simulink library "PhD_Library"  (R2018a)
settings: Solver=VariableStepAuto  StartTime=0.0  StopTime=10.0  RelTol=1e-3
values from neighbouring files (symbols this model uses):
  Ts = Ts_c    (= 1e-07)    [PlantStateEquations_abc_Script.m]
undefined symbols (not defined in the file or in its folder): D1, Delta, DiscIntNeverNeededParam, ESS, f_LPF_noise, fcutouti, fcutoutv, fn, fsw, Iap, Kp, PCC, Sn, tctrl, Ti, Ts_control, Ts_PWM, Uabp, Uanp, WT, X, zeta
libraries: $bdroot x84, powerlib_meascontrol x59, powerlib x56, peTransforms x32, cstblocks x2, simulink x2
(part 2 of 5)

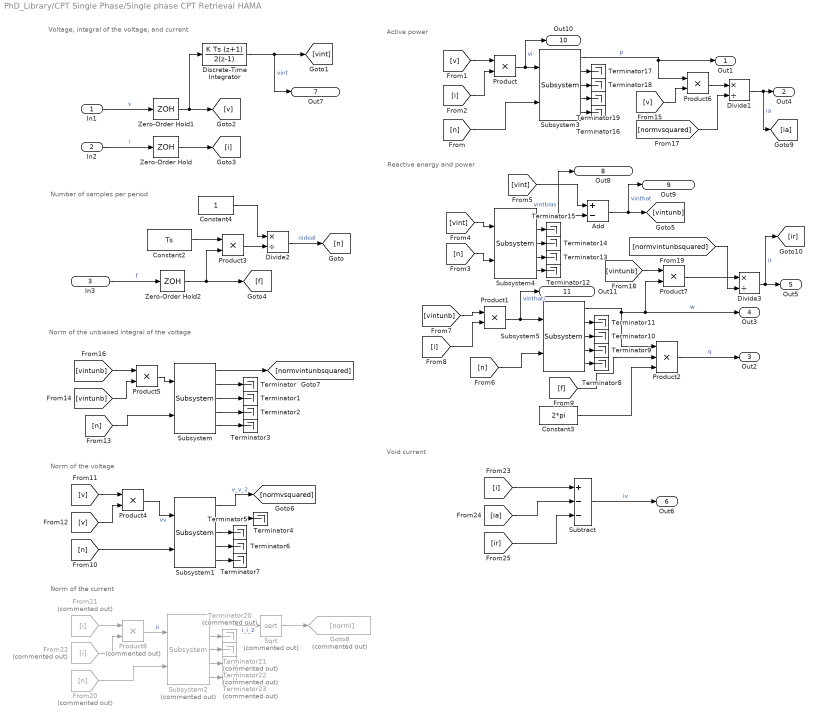
== system PhD_Library/CPT Single Phase/Single phase CPT Retrieval HAMA ==
  note: Void current
  note: Number of samples per period
  note: Norm of the voltage
  note: Voltage, integral of the voltage, and current
  note: Reactive energy and power
  note: Active power
  note: Norm of the current
  note: Norm of the unbiased integral of the voltage
  In1 : Inport
  In2 : Inport  Port=2
  In3 : Inport  Port=3
  Add : Sum  Inputs=+-
  Constant2 : Constant  Value=Ts
  Constant3 : Constant  Value=2*pi
  Constant4 : Constant
  Discrete-Time Integrator : DiscreteIntegrator  IntegratorMethod=Integration: Trapezoidal  SampleTime=Ts  ICPrevOutput=DiscIntNeverNeededParam  ICPrevScaledInput=DiscIntNeverNeededParam
  Divide1 : Product  Inputs=*/
  Divide2 : Product  Inputs=*/
  Divide3 : Product  Inputs=*/
  From20 : From  Commented=on  GotoTag=n
  From21 : From  Commented=on  GotoTag=i
  From22 : From  Commented=on  GotoTag=i
  Goto8 : Goto  Commented=on  GotoTag=normi
  Product{,1,3..7} (7 alike) : Product
  Product2 : Product  Inputs=3
  Product8 : Product  Commented=on
  Sqrt : Sqrt  Commented=on  SaturateOnIntegerOverflow=on
  Subsystem{,1,3..5} (5 alike) : $bdroot/Adaptive Moving Averages/Subsystem  NbSize=NbSize  Ts=Ts
  Subsystem2 : $bdroot/Adaptive Moving Averages/Subsystem  Commented=on  NbSize=NbSize  Ts=Ts
  Subtract : Sum  Inputs=+--
  Terminator{,1..19} (20 alike) : Terminator
  Terminator{20..23} (4 alike) : Terminator  Commented=on
  Zero-Order Hold : ZeroOrderHold  SampleTime=Ts
  Zero-Order Hold1 : ZeroOrderHold  SampleTime=Ts
  Zero-Order Hold2 : ZeroOrderHold  SampleTime=Ts
  Out1 : Outport
  Out4 : Outport  Port=2
  Out2 : Outport  Port=3
  Out3 : Outport  Port=4
  Out5 : Outport  Port=5
  Out6 : Outport  Port=6
  Out7 : Outport  Port=7
  Out8 : Outport  Port=8
  Out9 : Outport  Port=9
  Out10 : Outport  Port=10
  Out11 : Outport  Port=11
  wires:
  Product6/1 -> Divide1/1
  [i] -> Product/2
  Product3/1 -> Divide2/2
  Product7/1 -> Divide3/1
  [ia] -> Subtract/2
  [f] -> Product2/2
  Divide3/1 -> [ir], Out5/1  "ir"
  Subsystem2/1 -> Sqrt/1  "i_i_2"
  Product8/1 -> Subsystem2/1  "ii"
  [v] -> Product4/1
  Subtract/1 -> Out6/1  "iv"
  In2/1 -> Zero-Order Hold/1  "i"
  In1/1 -> Zero-Order Hold1/1  "v"
  [v] -> Product/1
  [v] -> Product4/2
  [n] -> Subsystem/2
  [vint] -> Add/1
  Add/1 -> Out9/1, [vintunb]  "vinthat"
  From21/1 -> Product8/1
  Subsystem4/1 -> Out8/1, Add/2  "vintbias"
  Zero-Order Hold2/1 -> Product3/2, [f]
  [ir] -> Subtract/3
  Divide2/1 -> [n]  "nideal"
  Product1/1 -> Subsystem5/1, Out11/1  "vinthati"
  Zero-Order Hold/1 -> [i]
  Divide1/1 -> [ia], Out4/1  "ia"
  [vintunb] -> Product7/1
  Product2/1 -> Out2/1  "q"
  Constant3/1 -> Product2/3
  From22/1 -> Product8/2
  [vintunb] -> Product5/1
  [normvintunbsquared] -> Divide3/2
  Discrete-Time Integrator/1 -> Out7/1, [vint]  "vint"
  [vintunb] -> Product5/2
  [i] -> Subtract/1
  Product5/1 -> Subsystem/1
  [vintunb] -> Product1/1
  Subsystem1/1 -> [normvsquared]  "v_v_2"
  Product/1 -> Subsystem3/1, Out10/1  "vi"
  [v] -> Product6/2
  Constant2/1 -> Product3/1
  [i] -> Product1/2
  Product4/1 -> Subsystem1/1  "vv"
  [n] -> Subsystem1/2
  Subsystem5/1 -> Product2/1, Product7/2, Out3/1  "w"
  [normvsquared] -> Divide1/2
  Zero-Order Hold1/1 -> [v], Discrete-Time Integrator/1
  In3/1 -> Zero-Order Hold2/1  "f"
  Constant4/1 -> Divide2/1
  Subsystem/1 -> [normvintunbsquared]
  Sqrt/1 -> Goto8/1
  Subsystem3/1 -> Product6/1, Out1/1  "p"
  From20/1 -> Subsystem2/2
  [n] -> Subsystem3/2
  [vint] -> Subsystem4/1
  [n] -> Subsystem4/2
  [n] -> Subsystem5/2
  Subsystem/2 -> Terminator/1
  Subsystem/3 -> Terminator1/1
  Subsystem/4 -> Terminator2/1
  Subsystem/5 -> Terminator3/1
  Subsystem1/2 -> Terminator4/1
  Subsystem1/3 -> Terminator5/1
  Subsystem1/4 -> Terminator6/1
  Subsystem1/5 -> Terminator7/1
  Subsystem5/5 -> Terminator8/1
  Subsystem5/4 -> Terminator9/1
  Subsystem5/3 -> Terminator10/1
  Subsystem5/2 -> Terminator11/1
  Subsystem4/5 -> Terminator12/1
  Subsystem4/4 -> Terminator13/1
  Subsystem4/3 -> Terminator14/1
  Subsystem4/2 -> Terminator15/1
  Subsystem3/5 -> Terminator16/1
  Subsystem3/2 -> Terminator17/1
  Subsystem3/3 -> Terminator18/1
  Subsystem3/4 -> Terminator19/1
  Subsystem2/2 -> Terminator20/1
  Subsystem2/3 -> Terminator21/1
  Subsystem2/4 -> Terminator22/1
  Subsystem2/5 -> Terminator23/1

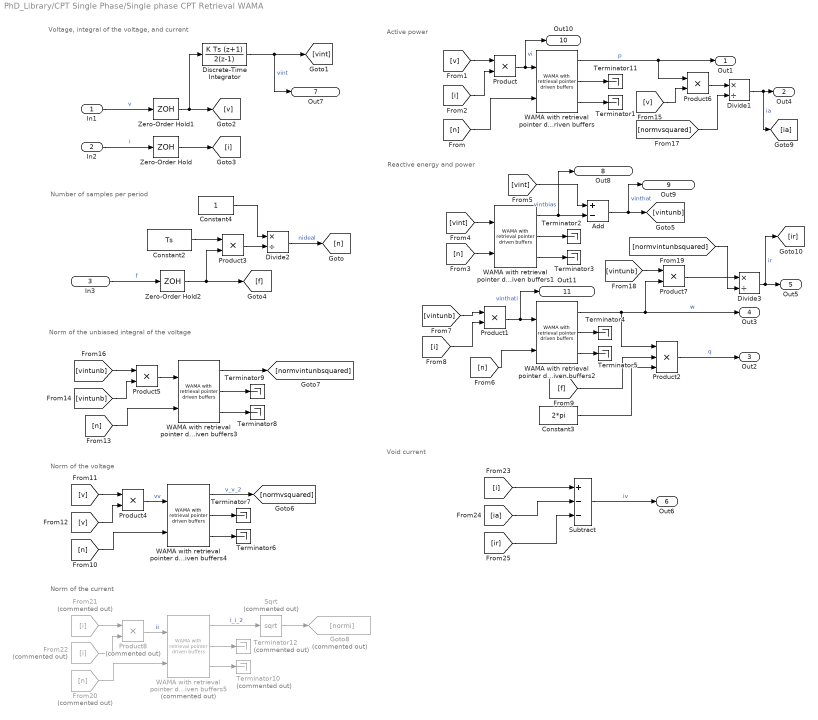
== system PhD_Library/CPT Single Phase/Single phase CPT Retrieval WAMA ==
  note: Voltage, integral of the voltage, and current
  note: Number of samples per period
  note: Reactive energy and power
  note: Active power
  note: Norm of the voltage
  note: Norm of the unbiased integral of the voltage
  note: Norm of the current
  note: Void current
  In1 : Inport
  In2 : Inport  Port=2
  In3 : Inport  Port=3
  Add : Sum  Inputs=+-
  Constant2 : Constant  Value=Ts
  Constant3 : Constant  Value=2*pi
  Constant4 : Constant
  Discrete-Time Integrator : DiscreteIntegrator  IntegratorMethod=Integration: Trapezoidal  SampleTime=Ts  ICPrevOutput=DiscIntNeverNeededParam  ICPrevScaledInput=DiscIntNeverNeededParam
  Divide1 : Product  Inputs=*/
  Divide2 : Product  Inputs=*/
  Divide3 : Product  Inputs=*/
  From20 : From  Commented=on  GotoTag=n
  From21 : From  Commented=on  GotoTag=i
  From22 : From  Commented=on  GotoTag=i
  Goto8 : Goto  Commented=on  GotoTag=normi
  Product{,1,3..7} (7 alike) : Product
  Product2 : Product  Inputs=3
  Product8 : Product  Commented=on
  Sqrt : Sqrt  Commented=on  SaturateOnIntegerOverflow=on
  Subtract : Sum  Inputs=+--
  Terminator{1..9,11} (10 alike) : Terminator
  Terminator10 : Terminator  Commented=on
  Terminator12 : Terminator  Commented=on
  WAMA with retrieval pointer driven buffers{,1..4} (5 alike) : $bdroot/Adaptive Moving Averages/WAMA with retrieval pointer driven buffers  NbSize=NbSize  Ts=Ts
  WAMA with retrieval pointer driven buffers5 : $bdroot/Adaptive Moving Averages/WAMA with retrieval pointer driven buffers  Commented=on  NbSize=NbSize  Ts=Ts
  Zero-Order Hold : ZeroOrderHold  SampleTime=Ts
  Zero-Order Hold1 : ZeroOrderHold  SampleTime=Ts
  Zero-Order Hold2 : ZeroOrderHold  SampleTime=Ts
  Out1 : Outport
  Out4 : Outport  Port=2
  Out2 : Outport  Port=3
  Out3 : Outport  Port=4
  Out5 : Outport  Port=5
  Out6 : Outport  Port=6
  Out7 : Outport  Port=7
  Out8 : Outport  Port=8
  Out9 : Outport  Port=9
  Out10 : Outport  Port=10
  Out11 : Outport  Port=11
  wires:
  Discrete-Time Integrator/1 -> Out7/1, [vint]  "vint"
  In3/1 -> Zero-Order Hold2/1  "f"
  Zero-Order Hold1/1 -> [v], Discrete-Time Integrator/1
  [i] -> Subtract/1
  WAMA with retrieval pointer driven buffers3/1 -> [normvintunbsquared]
  Product5/1 -> WAMA with retrieval pointer driven buffers3/1
  WAMA with retrieval pointer driven buffers3/2 -> Terminator9/1
  WAMA with retrieval pointer driven buffers3/3 -> Terminator8/1
  Product4/1 -> WAMA with retrieval pointer driven buffers4/1  "vv"
  WAMA with retrieval pointer driven buffers4/3 -> Terminator6/1
  WAMA with retrieval pointer driven buffers4/2 -> Terminator7/1
  WAMA with retrieval pointer driven buffers4/1 -> [normvsquared]  "v_v_2"
  [n] -> WAMA with retrieval pointer driven buffers4/2
  [vint] -> WAMA with retrieval pointer driven buffers1/1
  WAMA with retrieval pointer driven buffers5/3 -> Terminator10/1
  WAMA with retrieval pointer driven buffers1/2 -> Terminator2/1
  WAMA with retrieval pointer driven buffers/2 -> Terminator11/1
  WAMA with retrieval pointer driven buffers/3 -> Terminator1/1
  WAMA with retrieval pointer driven buffers2/2 -> Terminator4/1
  Product1/1 -> Out11/1, WAMA with retrieval pointer driven buffers2/1  "vinthati"
  [v] -> Product6/2
  WAMA with retrieval pointer driven buffers2/1 -> Product7/2, Out3/1, Product2/1  "w"
  Product/1 -> Out10/1, WAMA with retrieval pointer driven buffers/1  "vi"
  [vintunb] -> Product7/1
  [normvsquared] -> Divide1/2
  [normvintunbsquared] -> Divide3/2
  Divide1/1 -> [ia], Out4/1  "ia"
  Zero-Order Hold/1 -> [i]
  [vint] -> Add/1
  Constant3/1 -> Product2/3
  [i] -> Product1/2
  [vintunb] -> Product1/1
  Constant2/1 -> Product3/1
  [vintunb] -> Product5/1
  [ir] -> Subtract/3
  From22/1 -> Product8/2
  [n] -> WAMA with retrieval pointer driven buffers2/2
  WAMA with retrieval pointer driven buffers5/2 -> Terminator12/1
  Zero-Order Hold2/1 -> Product3/2, [f]
  Product7/1 -> Divide3/1
  WAMA with retrieval pointer driven buffers1/3 -> Terminator3/1
  Sqrt/1 -> Goto8/1
  Divide2/1 -> [n]  "nideal"
  WAMA with retrieval pointer driven buffers5/1 -> Sqrt/1  "i_i_2"
  Constant4/1 -> Divide2/1
  Product2/1 -> Out2/1  "q"
  [n] -> WAMA with retrieval pointer driven buffers3/2
  Product3/1 -> Divide2/2
  [n] -> WAMA with retrieval pointer driven buffers/2
  From20/1 -> WAMA with retrieval pointer driven buffers5/2
  [vintunb] -> Product5/2
  [v] -> Product4/2
  Product8/1 -> WAMA with retrieval pointer driven buffers5/1  "ii"
  Product6/1 -> Divide1/1
  WAMA with retrieval pointer driven buffers1/1 -> Out8/1, Add/2  "vintbias"
  Add/1 -> Out9/1, [vintunb]  "vinthat"
  [f] -> Product2/2
  In1/1 -> Zero-Order Hold1/1  "v"
  From21/1 -> Product8/1
  WAMA with retrieval pointer driven buffers/1 -> Product6/1, Out1/1  "p"
  Subtract/1 -> Out6/1  "iv"
  [i] -> Product/2
  In2/1 -> Zero-Order Hold/1  "i"
  [n] -> WAMA with retrieval pointer driven buffers1/2
  Divide3/1 -> [ir], Out5/1  "ir"
  [v] -> Product4/1
  WAMA with retrieval pointer driven buffers2/3 -> Terminator5/1
  [v] -> Product/1
  [ia] -> Subtract/2

== system PhD_Library/Offshore_Oil_and_Wind/Balanced_3_phase_Vsource ==
  amp_pu : Inport
  time_s : Inport  Port=2
  phase_deg : Inport  Port=3
  pos1_neg-1 : Inport  Port=4
  f_pu : Inport  Port=5
  Add3 : Sum  Inputs=+-+
  Add4 : Sum  Inputs=+++
  Add5 : Sum
  Amplitude_Base : Constant  Value=BaseAmp
  Bus Creator : BusCreator  Inputs=3
  Constant : Constant  Value=2*pi
  Constant4 : Constant  Value=2*pi/3
  Constant6 : Constant  Value=2*pi
  Controlled Voltage Source : powerlib/Electrical Sources/Controlled Voltage Source  Initialize=off  Source_Type=AC  Amplitude=ESS.LSC.Ub*(2/3)^0.5  Phase=0  Frequency=PCC.fn  Measurements=None
  Controlled Voltage Source1 : powerlib/Electrical Sources/Controlled Voltage Source  Initialize=off  Source_Type=AC  Amplitude=ESS.LSC.Ub*(2/3)^0.5  Phase=-120  Frequency=PCC.fn  Measurements=None
  Controlled Voltage Source2 : powerlib/Electrical Sources/Controlled Voltage Source  Initialize=off  Source_Type=AC  Amplitude=ESS.LSC.Ub*(2/3)^0.5  Phase=120  Frequency=PCC.fn  Measurements=None
  Gain : Gain  Gain=pi/180
  Gain1 : Gain  Gain=fn
  Mux : Mux  Inputs=3
  Product{1,3..8} (7 alike) : Product
  Product2 : Product  Inputs=3
  Relay : Relay  OnSwitchValue=0  OffSwitchValue=-0.1  OffOutputValue=-1
  Trigonometric Function3 : Trigonometry
  Trigonometric Function4 : Trigonometry
  Trigonometric Function5 : Trigonometry
  mod : Math  Operator=mod  SaturateOnIntegerOverflow=on
  Va+ : PMIOPort  Side=Right
  Vb+ : PMIOPort  Port=2  Side=Right
  Vc+ : PMIOPort  Port=3  Side=Right
  Va- : PMIOPort  Port=4  Side=Right
  Vb- : PMIOPort  Port=5  Side=Right
  Vc- : PMIOPort  Port=6  Side=Right
  Amp_V : Outport
  phase_rad : Outport  Port=2
  wt_phase_abc : Outport  Port=3
  Vabc : Outport  Port=4
  wires:
  Add4/1 -> Mux/3, Trigonometric Function5/1
  Product6/1 -> phase_rad/1, Add4/3, Add3/3, Add5/2  "phase"
  Add3/1 -> Mux/2, Trigonometric Function4/1
  pos1_neg-1/1 -> Relay/1
  Product3/1 -> Bus Creator/1, Controlled Voltage Source/1  "Va"
  amp_pu/1 -> Product1/1
  Product8/1 -> Add3/2, Add4/2
  Product5/1 -> Bus Creator/3, Controlled Voltage Source2/1  "Vc"
  Product4/1 -> Bus Creator/2, Controlled Voltage Source1/1  "Vb"
  Amplitude_Base/1 -> Product1/2
  Product7/1 -> Product8/1
  Product1/1 -> Product5/1, Product4/1, Product3/1, Amp_V/1  "amp"
  Relay/1 -> Product8/2
  Trigonometric Function3/1 -> Product3/2
  Product2/1 -> Add5/1, Add4/1, Add3/1  "wt"
  Trigonometric Function5/1 -> Product5/2
  Add5/1 -> Mux/1, Trigonometric Function3/1
  Trigonometric Function4/1 -> Product4/2
  phase_deg/1 -> Gain/1
  time_s/1 -> Product2/2
  Constant/1 -> Product2/1
  Gain1/1 -> Product2/3
  Bus Creator/1 -> Vabc/1
  Constant6/1 -> mod/2
  mod/1 -> wt_phase_abc/1
  Gain/1 -> Product6/1  "phase"
  Constant4/1 -> Product7/2
  Mux/1 -> mod/1
  f_pu/1 -> Product7/1, Product6/2, Gain1/1
  connections:
  Vb+/RConn1 -- Controlled Voltage Source1/RConn1
  Vc+/RConn1 -- Controlled Voltage Source2/RConn1
  Va+/RConn1 -- Controlled Voltage Source/RConn1
  Va-/RConn1 -- Controlled Voltage Source/LConn1
  Vb-/RConn1 -- Controlled Voltage Source1/LConn1
  Vc-/RConn1 -- Controlled Voltage Source2/LConn1

== system PhD_Library/Offshore_Oil_and_Wind/Digital first order LPF ==
  note: Transfer function: alpha / ( 1 + ( alpha -1 ) z^{-1} )
  note: alpha = Ts / ( 1/(2 pi fcutout) + Ts )
  note: y = alpha x + ( 1 - alpha) y z^{-1}
  in : Inport
  Add7 : Sum  Commented=on  Inputs=+-
  Discrete Filter : DiscreteFilter  Numerator=[Ts/(1/(2*pi*fcutout)+Ts)]  Denominator=[1 Ts/(1/(2*pi*fcutout)+Ts)-1]  SampleTime=Ts
  Discrete-Time Integrator : DiscreteIntegrator  Commented=on  IntegratorMethod=Integration: Trapezoidal  SampleTime=Ts  ICPrevOutput=DiscIntNeverNeededParam  ICPrevScaledInput=DiscIntNeverNeededParam
  Gain6 : Gain  Commented=on  Gain=2*pi*fcutout
  Rate Transition3 : RateTransition  OutPortSampleTime=Ts
  out : Outport
  wires:
  Add7/1 -> Gain6/1
  Discrete-Time Integrator/1 -> Add7/2
  in/1 -> Rate Transition3/1
  Gain6/1 -> Discrete-Time Integrator/1
  Rate Transition3/1 -> Add7/1, Discrete Filter/1
  Discrete Filter/1 -> out/1

== system PhD_Library/Offshore_Oil_and_Wind/DualRegulator ==
  idqref : Inport
  vabc : Inport  Port=2
  iabc : Inport  Port=3
  wt : Inport  Port=4
  w_pu : Inport  Port=5
  Udc : Inport  Port=6
  1=enable_acb : Inport  Port=7
  1=no,2=Notch,3=DSC : Inport  Port=8
  pre_mult_PI_errors : Inport  Port=9
  force_int : Inport  Port=10
  force_val : Inport  Port=11
  Bus Creator : BusCreator  Inputs=4
  Constant1 : Constant  Value=0
  Constant10 : Constant
  Constant14 : Constant
  Constant18 : Constant  Value=[0 0]
  Constant6 : Constant
  Constant8 : Constant  Value=0
  Idq_Dec_Signs_Fdbk_Ref : $bdroot/Offshore_Oil_and_Wind/Idq_Dec_Signs_Fdbk_Ref  Ts=Ts  fn=fgrid  Kp=PI_Kp  Ti=PI_Ti  L=PI_X  PI_max=PI_max  PI_min=PI_min  TrafoPhaseComp=0
  Idq_Dec_Signs_Fdbk_Ref_acb : $bdroot/Offshore_Oil_and_Wind/Idq_Dec_Signs_Fdbk_Ref  Ts=Ts  fn=fgrid  Kp=PI_Kp  Ti=PI_Ti  L=PI_X  PI_max=PI_max  PI_min=PI_min  TrafoPhaseComp=0
  PWM_abc_negwt_acb : $bdroot/Offshore_Oil_and_Wind/PWM_abc_negwt_acb  fsw=PWM_fsw  Ts=PWM_Ts  Uabp=PWM_Uabp  PWM_Ini_Phase=PWM_Ini
  Selector1 : Selector  InputPortWidth=3  IndexOptions=Index vector (dialog)  Indices=[1 3 2]  OutputSizes=1
  Selector7 : Selector  InputPortWidth=3  IndexOptions=Index vector (dialog)  Indices=[1 3 2]  OutputSizes=1
  Terminator{1..4,24} (5 alike) : Terminator
  abc_dq_bypassnotch : $bdroot/Offshore_Oil_and_Wind/abc_dq_bypassnotch  Ts=Ts  fn=2*fgrid  fcutoutv=fcutoutLPF  fcutouti=fcutoutLPF  zeta=zetanotch
  abc_dq_bypassnotch1 : $bdroot/Offshore_Oil_and_Wind/abc_dq_bypassnotch  Ts=Ts  fn=2*fgrid  fcutoutv=fcutoutLPF  fcutouti=fcutoutLPF  zeta=zetanotch
  idqref_gen_for_cnst_p : $bdroot/Offshore_Oil_and_Wind/idqref_gen_for_cnst_p  Ts_control=Ts
  PWMpulses : Outport
  Uabcref : Outport  Port=2
  mvidq : Outport  Port=3
  mpi+ : Outport  Port=4
  mpi- : Outport  Port=5
  wires:
  Udc/1 -> PWM_abc_negwt_acb/7
  abc_dq_bypassnotch1/1 -> idqref_gen_for_cnst_p/2, Bus Creator/3, Idq_Dec_Signs_Fdbk_Ref_acb/2  "vdq-"
  [w_pu] -> Idq_Dec_Signs_Fdbk_Ref/4
  PWM_abc_negwt_acb/3 -> Terminator24/1
  Constant14/1 -> Idq_Dec_Signs_Fdbk_Ref_acb/5
  abc_dq_bypassnotch/1 -> idqref_gen_for_cnst_p/1, Bus Creator/1, Idq_Dec_Signs_Fdbk_Ref/2  "vdq+"
  abc_dq_bypassnotch1/2 -> Bus Creator/4, Idq_Dec_Signs_Fdbk_Ref_acb/3  "idq-"
  Constant10/1 -> PWM_abc_negwt_acb/2
  Constant8/1 -> PWM_abc_negwt_acb/4
  abc_dq_bypassnotch/2 -> Bus Creator/2, Idq_Dec_Signs_Fdbk_Ref/3  "idq+"
  1=enable_acb/1 -> PWM_abc_negwt_acb/6
  Idq_Dec_Signs_Fdbk_Ref/1 -> PWM_abc_negwt_acb/1
  PWM_abc_negwt_acb/1 -> PWMpulses/1
  PWM_abc_negwt_acb/2 -> Uabcref/1  "Uabcref"
  Constant6/1 -> Idq_Dec_Signs_Fdbk_Ref/5
  Constant1/1 -> Idq_Dec_Signs_Fdbk_Ref_acb/6, Idq_Dec_Signs_Fdbk_Ref/6
  vabc/1 -> abc_dq_bypassnotch/1, Selector7/1
  iabc/1 -> abc_dq_bypassnotch/2, Selector1/1
  Idq_Dec_Signs_Fdbk_Ref_acb/1 -> PWM_abc_negwt_acb/5
  wt/1 -> abc_dq_bypassnotch/3, abc_dq_bypassnotch1/3, [theta]
  Selector7/1 -> abc_dq_bypassnotch1/1
  Selector1/1 -> abc_dq_bypassnotch1/2
  Constant18/1 -> PWM_abc_negwt_acb/3
  idqref/1 -> idqref_gen_for_cnst_p/3, Idq_Dec_Signs_Fdbk_Ref/1
  idqref_gen_for_cnst_p/1 -> Idq_Dec_Signs_Fdbk_Ref_acb/1
  [theta] -> PWM_abc_negwt_acb/8
  1=no,2=Notch,3=DSC/1 -> abc_dq_bypassnotch/5, abc_dq_bypassnotch1/5
  Bus Creator/1 -> mvidq/1
  w_pu/1 -> abc_dq_bypassnotch/4, abc_dq_bypassnotch1/4, [w_pu]
  [w_pu] -> Idq_Dec_Signs_Fdbk_Ref_acb/4
  pre_mult_PI_errors/1 -> Idq_Dec_Signs_Fdbk_Ref_acb/7, Idq_Dec_Signs_Fdbk_Ref/7
  force_int/1 -> Idq_Dec_Signs_Fdbk_Ref_acb/8, Idq_Dec_Signs_Fdbk_Ref/8
  force_val/1 -> Idq_Dec_Signs_Fdbk_Ref_acb/10, Idq_Dec_Signs_Fdbk_Ref_acb/9, Idq_Dec_Signs_Fdbk_Ref/10, Idq_Dec_Signs_Fdbk_Ref/9
  Idq_Dec_Signs_Fdbk_Ref/4 -> mpi+/1
  Idq_Dec_Signs_Fdbk_Ref_acb/4 -> mpi-/1
  Idq_Dec_Signs_Fdbk_Ref/2 -> Terminator1/1
  Idq_Dec_Signs_Fdbk_Ref/3 -> Terminator2/1
  Idq_Dec_Signs_Fdbk_Ref_acb/2 -> Terminator3/1
  Idq_Dec_Signs_Fdbk_Ref_acb/3 -> Terminator4/1

== system PhD_Library/Offshore_Oil_and_Wind/Enabled ==
  En : Inport
  MATLAB Function : MATLAB Function  SystemSampleTime=Ts
      settings: RTWSystemCode=Inline
  Enabled : Outport
  Disabled : Outport  Port=2
  wires:
  En/1 -> MATLAB Function/1(En)
  MATLAB Function/1(Enabled) -> Enabled/1
  MATLAB Function/2(Disabled) -> Disabled/1

== system PhD_Library/Offshore_Oil_and_Wind/Garbage ==
  In1 : Inport
  In2 : Inport  Port=2
  Demux4 : Demux  Outputs=3
  Demux5 : Demux  Outputs=3
  Mux3 : Mux  Inputs=[1 1 1]
  Mux4 : Mux  Inputs=[1 1 1]
  Transfer Fcn : TransferFcn  Denominator=[1/(2*pi*fcutoutv) 1]
  Transfer Fcn1 : TransferFcn  Denominator=[1/(2*pi*fcutoutv) 1]
  Transfer Fcn2 : TransferFcn  Denominator=[1/(2*pi*fcutoutv) 1]
  Transfer Fcn3 : TransferFcn  Denominator=[1/(2*pi*fcutouti) 1]
  Transfer Fcn4 : TransferFcn  Denominator=[1/(2*pi*fcutouti) 1]
  Transfer Fcn5 : TransferFcn  Denominator=[1/(2*pi*fcutouti) 1]
  Out1 : Outport
  Out2 : Outport  Port=2
  wires:
  Demux5/1 -> Transfer Fcn3/1
  Transfer Fcn2/1 -> Mux3/3
  Demux4/1 -> Transfer Fcn/1
  Demux5/3 -> Transfer Fcn5/1
  Transfer Fcn3/1 -> Mux4/1
  Transfer Fcn4/1 -> Mux4/2
  Demux4/3 -> Transfer Fcn2/1
  Transfer Fcn5/1 -> Mux4/3
  Demux4/2 -> Transfer Fcn1/1
  Transfer Fcn/1 -> Mux3/1
  Mux3/1 -> Out2/1
  Transfer Fcn1/1 -> Mux3/2
  Demux5/2 -> Transfer Fcn4/1
  In1/1 -> Demux5/1
  Mux4/1 -> Out1/1
  In2/1 -> Demux4/1

== system PhD_Library/Offshore_Oil_and_Wind/Ideal3PhaseVoltSource ==
  amp_pu : Inport
  f_pu : Inport  Port=2
  phase_deg : Inport  Port=3
  pos1_neg-1 : Inport  Port=4
  Harm_nr : Inport  Port=5
  Add3 : Sum  Inputs=+-+
  Add4 : Sum  Inputs=+++
  Add5 : Sum
  Amplitude_Base : Constant  Value=BaseAmp
  Bus Creator : BusCreator  Inputs=3
  Constant : Constant  Value=2*pi
  Constant4 : Constant  Value=2*pi/3
  Constant6 : Constant  Value=2*pi
  Controlled Voltage Source : powerlib/Electrical Sources/Controlled Voltage Source  Initialize=off  Source_Type=AC  Amplitude=ESS.LSC.Ub*(2/3)^0.5  Phase=0  Frequency=PCC.fn  Measurements=None
  Controlled Voltage Source1 : powerlib/Electrical Sources/Controlled Voltage Source  Initialize=off  Source_Type=AC  Amplitude=ESS.LSC.Ub*(2/3)^0.5  Phase=-120  Frequency=PCC.fn  Measurements=None
  Controlled Voltage Source2 : powerlib/Electrical Sources/Controlled Voltage Source  Initialize=off  Source_Type=AC  Amplitude=ESS.LSC.Ub*(2/3)^0.5  Phase=120  Frequency=PCC.fn  Measurements=None
  Gain : Gain  Gain=pi/180
  Gain1 : Gain  Gain=fn
  Integrator : Integrator
  Mux : Mux  Inputs=3
  Product{1,3..8} (7 alike) : Product
  Product2 : Product  Inputs=3
  Relay : Relay  OnSwitchValue=0  OffSwitchValue=-0.1  OffOutputValue=-1
  Trigonometric Function3 : Trigonometry
  Trigonometric Function4 : Trigonometry
  Trigonometric Function5 : Trigonometry
  mod : Math  Operator=mod  SaturateOnIntegerOverflow=on
  Va+ : PMIOPort  Side=Right
  Vb+ : PMIOPort  Port=2  Side=Right
  Vc+ : PMIOPort  Port=3  Side=Right
  Va- : PMIOPort  Port=4  Side=Right
  Vb- : PMIOPort  Port=5  Side=Right
  Vc- : PMIOPort  Port=6  Side=Right
  Amp_V : Outport
  phase_rad : Outport  Port=2
  wt_phase_abc : Outport  Port=3
  Vabc : Outport  Port=4
  wires:
  Add4/1 -> Mux/3, Trigonometric Function5/1
  Product6/1 -> phase_rad/1, Add4/3, Add3/3, Add5/2  "phase"
  Add3/1 -> Mux/2, Trigonometric Function4/1
  pos1_neg-1/1 -> Relay/1
  Product3/1 -> Bus Creator/1, Controlled Voltage Source/1  "Va"
  amp_pu/1 -> Product1/1
  Product8/1 -> Add3/2, Add4/2
  Product5/1 -> Bus Creator/3, Controlled Voltage Source2/1  "Vc"
  Product4/1 -> Bus Creator/2, Controlled Voltage Source1/1  "Vb"
  Amplitude_Base/1 -> Product1/2
  Product7/1 -> Product8/1
  Product1/1 -> Product5/1, Product4/1, Product3/1, Amp_V/1  "amp"
  Relay/1 -> Product8/2
  Trigonometric Function3/1 -> Product3/2
  Product2/1 -> Add5/1, Add4/1, Add3/1  "wt"
  Trigonometric Function5/1 -> Product5/2
  Add5/1 -> Mux/1, Trigonometric Function3/1
  Trigonometric Function4/1 -> Product4/2
  phase_deg/1 -> Gain/1
  f_pu/1 -> Integrator/1
  Constant/1 -> Product2/1
  Gain1/1 -> Product2/3
  Bus Creator/1 -> Vabc/1
  Constant6/1 -> mod/2
  mod/1 -> wt_phase_abc/1
  Gain/1 -> Product6/1  "phase"
  Constant4/1 -> Product7/2
  Mux/1 -> mod/1
  Harm_nr/1 -> Product7/1, Product6/2, Gain1/1
  Integrator/1 -> Product2/2  "time"
  connections:
  Vb+/RConn1 -- Controlled Voltage Source1/RConn1
  Vc+/RConn1 -- Controlled Voltage Source2/RConn1
  Va+/RConn1 -- Controlled Voltage Source/RConn1
  Va-/RConn1 -- Controlled Voltage Source/LConn1
  Vb-/RConn1 -- Controlled Voltage Source1/LConn1
  Vc-/RConn1 -- Controlled Voltage Source2/LConn1

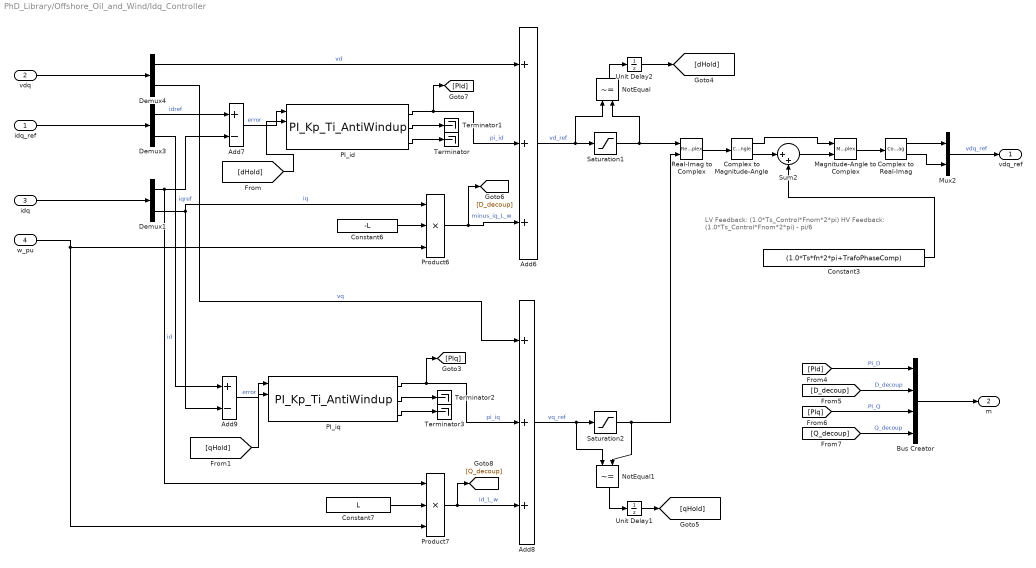
== system PhD_Library/Offshore_Oil_and_Wind/Idq_Controller ==
  note: LV Feedback: (1.0*Ts_Control*Fnom*2*pi)
      | HV Feedback: (1.0*Ts_Control*Fnom*2*pi) - pi/6
  idq_ref : Inport
  vdq : Inport  Port=2
  idq : Inport  Port=3
  w_pu : Inport  Port=4
  Add6 : Sum  Inputs=+++
  Add7 : Sum  Inputs=+-
  Add8 : Sum  Inputs=+++
  Add9 : Sum  Inputs=+-
  Bus Creator : BusCreator  Inputs=4
  Complex to Magnitude-Angle : ComplexToMagnitudeAngle
  Complex to Real-Imag : ComplexToRealImag
  Constant3 : Constant  Value=(1.0*Ts*fn*2*pi+TrafoPhaseComp)  SampleTime=Ts
  Constant6 : Constant  Value=-L  SampleTime=Ts
  Constant7 : Constant  Value=L  SampleTime=Ts
  Demux1 : Demux  Outputs=2
  Demux3 : Demux  Outputs=2
  Demux4 : Demux  Outputs=2
  Magnitude-Angle to Complex : MagnitudeAngleToComplex
  Mux2 : Mux  Inputs=2
  NotEqual : RelationalOperator  Operator=~=  OutDataTypeStr=boolean  RndMeth=Simplest
  NotEqual1 : RelationalOperator  Operator=~=  OutDataTypeStr=boolean  RndMeth=Simplest
  PI_id : $bdroot/Offshore_Oil_and_Wind/PI_Kp_Ti_AntiWindup  Ts=Ts  Kp=Kp  Ti=Ti  PI_max=PI_max  PI_min=PI_min
  PI_iq : $bdroot/Offshore_Oil_and_Wind/PI_Kp_Ti_AntiWindup  Ts=Ts  Kp=Kp  Ti=Ti  PI_max=PI_max  PI_min=PI_min
  Product6 : Product  Inputs=3  RndMeth=Zero
  Product7 : Product  Inputs=3  RndMeth=Zero
  Real-Imag to Complex : RealImagToComplex
  Saturation1 : Saturate  UpperLimit=PI_max  LowerLimit=PI_min
  Saturation2 : Saturate  UpperLimit=PI_max  LowerLimit=PI_min
  Sum2 : Sum  Inputs=|++
  Terminator{,1..3} (4 alike) : Terminator
  Unit Delay1 : UnitDelay  SampleTime=Ts
  Unit Delay2 : UnitDelay  SampleTime=Ts
  vdq_ref : Outport
  m : Outport  Port=2
  wires:
  PI_iq/1 -> [PIq], Add8/2  "pi_iq"
  PI_iq/2 -> Terminator2/1
  PI_id/2 -> Terminator1/1
  w_pu/1 -> Product7/3, Product6/3
  Add9/1 -> PI_iq/1  "error"
  PI_id/1 -> [PId], Add6/2  "pi_id"
  Constant6/1 -> Product6/2
  Constant7/1 -> Product7/2
  Demux1/1 -> Add7/2, Product7/1  "id"
  Product7/1 -> [Q_decoup], Add8/3  "id_L_w"
  Demux4/1 -> Add6/1  "vd"
  Add7/1 -> PI_id/1  "error"
  Demux1/2 -> Product6/1, Add9/2  "iq"
  Product6/1 -> [D_decoup], Add6/3  "minus_iq_L_w"
  PI_iq/3 -> Terminator3/1
  PI_id/3 -> Terminator/1
  Demux4/2 -> Add8/1  "vq"
  Mux2/1 -> vdq_ref/1  "vdq_ref"
  idq/1 -> Demux1/1
  vdq/1 -> Demux4/1
  Add8/1 -> NotEqual1/1, Saturation2/1  "vq_ref"
  Add6/1 -> NotEqual/1, Saturation1/1  "vd_ref"
  idq_ref/1 -> Demux3/1
  Demux3/1 -> Add7/1  "idref"
  Demux3/2 -> Add9/1  "iqref"
  Magnitude-Angle to Complex/1 -> Complex to Real-Imag/1
  Real-Imag to Complex/1 -> Complex to Magnitude-Angle/1
  Complex to Magnitude-Angle/1 -> Magnitude-Angle to Complex/1
  Complex to Magnitude-Angle/2 -> Sum2/1
  Sum2/1 -> Magnitude-Angle to Complex/2
  Constant3/1 -> Sum2/2
  Complex to Real-Imag/1 -> Mux2/1
  Complex to Real-Imag/2 -> Mux2/2
  [PId] -> Bus Creator/1  "PI_D"
  [D_decoup] -> Bus Creator/2  "D_decoup"
  [PIq] -> Bus Creator/3  "PI_Q"
  Bus Creator/1 -> m/1
  [Q_decoup] -> Bus Creator/4  "Q_decoup"
  Saturation1/1 -> NotEqual/2, Real-Imag to Complex/1
  NotEqual/1 -> Unit Delay2/1
  Saturation2/1 -> NotEqual1/2, Real-Imag to Complex/2
  NotEqual1/1 -> Unit Delay1/1
  Unit Delay2/1 -> [dHold]
  Unit Delay1/1 -> [qHold]
  [dHold] -> PI_id/2
  [qHold] -> PI_iq/2

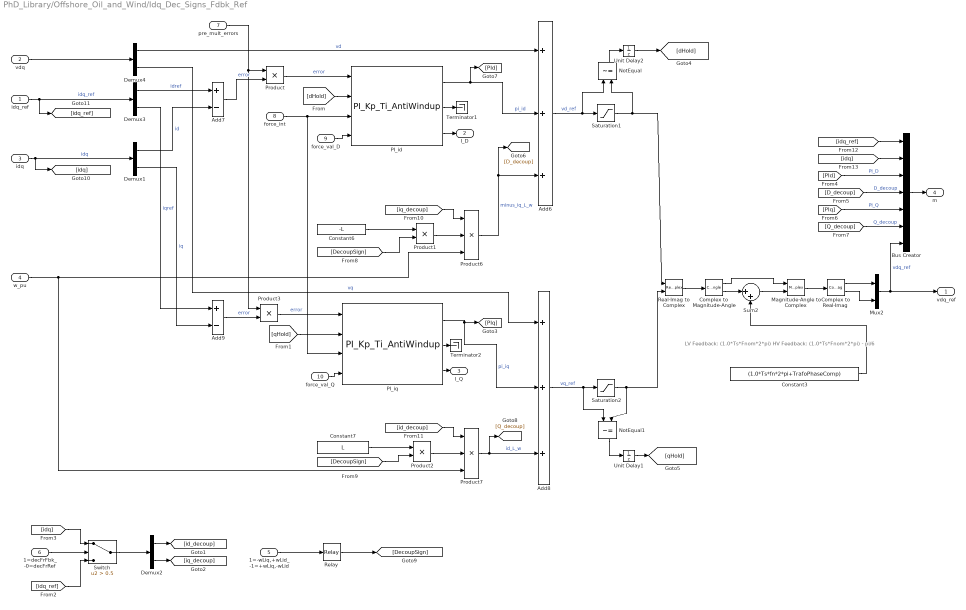
== system PhD_Library/Offshore_Oil_and_Wind/Idq_Dec_Signs_Fdbk_Ref ==
  note: LV Feedback: (1.0*Ts*Fnom*2*pi)
      | HV Feedback: (1.0*Ts*Fnom*2*pi) - pi/6
  idq_ref : Inport
  vdq : Inport  Port=2
  idq : Inport  Port=3
  w_pu : Inport  Port=4
  1=-wLiq,+wLid_-1=+wLiq,-wLid : Inport  Port=5
  1=decFrFbk_-0=decFrRef : Inport  Port=6
  pre_mult_errors : Inport  Port=7
  force_int : Inport  Port=8
  force_val_D : Inport  Port=9
  force_val_Q : Inport  Port=10
  Add6 : Sum  Inputs=+++
  Add7 : Sum  Inputs=+-
  Add8 : Sum  Inputs=+++
  Add9 : Sum  Inputs=+-
  Bus Creator : BusCreator  Inputs=7
  Complex to Magnitude-Angle : ComplexToMagnitudeAngle
  Complex to Real-Imag : ComplexToRealImag
  Constant3 : Constant  Value=(1.0*Ts*fn*2*pi+TrafoPhaseComp)  SampleTime=Ts
  Constant6 : Constant  Value=-L  SampleTime=Ts
  Constant7 : Constant  Value=L  SampleTime=Ts
  Demux{1..4} (4 alike) : Demux  Outputs=2
  Magnitude-Angle to Complex : MagnitudeAngleToComplex
  Mux2 : Mux  Inputs=2
  NotEqual : RelationalOperator  Operator=~=  OutDataTypeStr=boolean  RndMeth=Simplest
  NotEqual1 : RelationalOperator  Operator=~=  OutDataTypeStr=boolean  RndMeth=Simplest
  PI_id : $bdroot/Offshore_Oil_and_Wind/PI_Kp_Ti_AntiWindup  Ts=Ts  Kp=Kp  Ti=Ti  PI_max=PI_max  PI_min=PI_min
  PI_iq : $bdroot/Offshore_Oil_and_Wind/PI_Kp_Ti_AntiWindup  Ts=Ts  Kp=Kp  Ti=Ti  PI_max=PI_max  PI_min=PI_min
  Product : Product
  Product1 : Product  RndMeth=Zero
  Product2 : Product  RndMeth=Zero
  Product3 : Product
  Product6 : Product  Inputs=3  RndMeth=Zero
  Product7 : Product  Inputs=3  RndMeth=Zero
  Real-Imag to Complex : RealImagToComplex
  Relay : Relay  OnSwitchValue=0  OffSwitchValue=-0.1  OffOutputValue=-1
  Saturation1 : Saturate  UpperLimit=PI_max  LowerLimit=PI_min
  Saturation2 : Saturate  UpperLimit=PI_max  LowerLimit=PI_min
  Sum2 : Sum  Inputs=|++
  Switch : Switch  Criteria=u2 > Threshold  Threshold=0.5
  Terminator1 : Terminator
  Terminator2 : Terminator
  Unit Delay1 : UnitDelay  SampleTime=Ts
  Unit Delay2 : UnitDelay  SampleTime=Ts
  vdq_ref : Outport
  I_D : Outport  Port=2
  I_Q : Outport  Port=3
  m : Outport  Port=4
  wires:
  PI_iq/1 -> Add8/2, [PIq]  "pi_iq"
  PI_iq/2 -> Terminator2/1
  PI_id/2 -> Terminator1/1
  w_pu/1 -> Product7/3, Product6/3
  Product3/1 -> PI_iq/1  "error"
  PI_id/1 -> Add6/2, [PId]  "pi_id"
  Constant6/1 -> Product1/1
  Constant7/1 -> Product2/1
  Demux1/1 -> Add7/2  "id"
  Product7/1 -> [Q_decoup], Add8/3  "id_L_w"
  Demux4/1 -> Add6/1  "vd"
  Product/1 -> PI_id/1  "error"
  Demux1/2 -> Add9/2  "iq"
  Product6/1 -> [D_decoup], Add6/3  "minus_iq_L_w"
  PI_iq/3 -> I_Q/1
  PI_id/3 -> I_D/1
  Demux4/2 -> Add8/1  "vq"
  Mux2/1 -> Bus Creator/7, vdq_ref/1  "vdq_ref"
  idq/1 -> [idq], Demux1/1  "idq"
  vdq/1 -> Demux4/1
  Add8/1 -> NotEqual1/1, Saturation2/1  "vq_ref"
  Add6/1 -> NotEqual/1, Saturation1/1  "vd_ref"
  idq_ref/1 -> [idq_ref], Demux3/1  "idq_ref"
  Demux3/1 -> Add7/1  "idref"
  Demux3/2 -> Add9/1  "iqref"
  Magnitude-Angle to Complex/1 -> Complex to Real-Imag/1
  Real-Imag to Complex/1 -> Complex to Magnitude-Angle/1
  Complex to Magnitude-Angle/1 -> Magnitude-Angle to Complex/1
  Complex to Magnitude-Angle/2 -> Sum2/1
  Sum2/1 -> Magnitude-Angle to Complex/2
  Constant3/1 -> Sum2/2
  Complex to Real-Imag/1 -> Mux2/1
  Complex to Real-Imag/2 -> Mux2/2
  [PId] -> Bus Creator/3  "PI_D"
  [D_decoup] -> Bus Creator/4  "D_decoup"
  [PIq] -> Bus Creator/5  "PI_Q"
  Bus Creator/1 -> m/1
  [Q_decoup] -> Bus Creator/6  "Q_decoup"
  Saturation1/1 -> NotEqual/2, Real-Imag to Complex/1
  NotEqual/1 -> Unit Delay2/1
  Saturation2/1 -> NotEqual1/2, Real-Imag to Complex/2
  NotEqual1/1 -> Unit Delay1/1
  Unit Delay2/1 -> [dHold]
  Unit Delay1/1 -> [qHold]
  [dHold] -> PI_id/2
  [qHold] -> PI_iq/2
  Relay/1 -> [DecoupSign]
  1=-wLiq,+wLid_-1=+wLiq,-wLid/1 -> Relay/1
  [DecoupSign] -> Product1/2
  Product1/1 -> Product6/2
  Product2/1 -> Product7/2
  [DecoupSign] -> Product2/2
  [idq_ref] -> Switch/3
  Demux2/2 -> [iq_decoup]
  1=decFrFbk_-0=decFrRef/1 -> Switch/2
  Demux2/1 -> [id_decoup]
  Switch/1 -> Demux2/1
  [idq] -> Switch/1
  [iq_decoup] -> Product6/1
  [id_decoup] -> Product7/1
  [idq_ref] -> Bus Creator/1
  [idq] -> Bus Creator/2
  force_int/1 -> PI_iq/3, PI_id/3
  force_val_D/1 -> PI_id/4
  force_val_Q/1 -> PI_iq/4
  Add9/1 -> Product3/2  "error"
  Add7/1 -> Product/2  "error"
  pre_mult_errors/1 -> Product3/1, Product/1

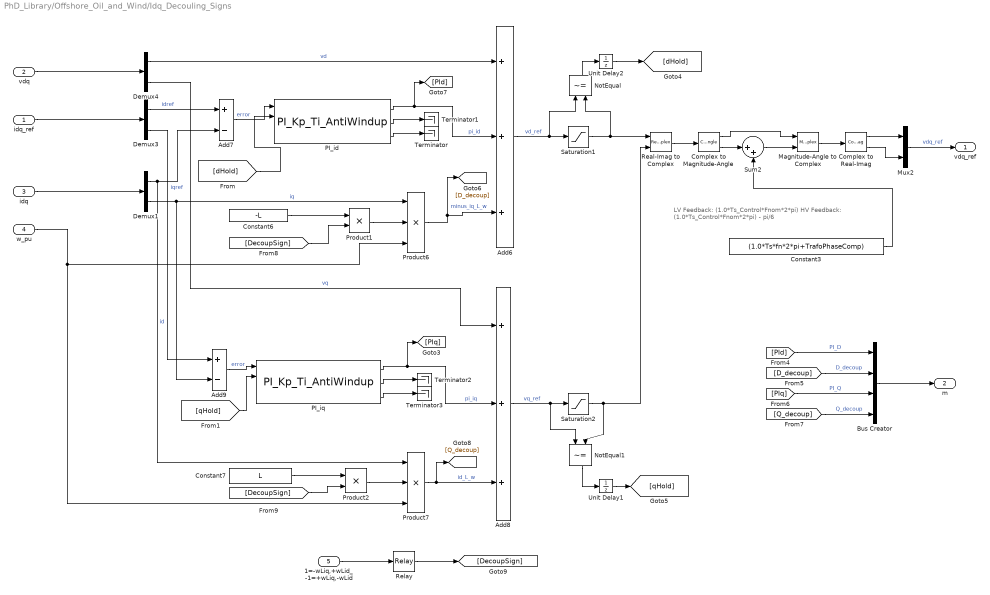
== system PhD_Library/Offshore_Oil_and_Wind/Idq_Decouling_Signs ==
  note: LV Feedback: (1.0*Ts_Control*Fnom*2*pi)
      | HV Feedback: (1.0*Ts_Control*Fnom*2*pi) - pi/6
  idq_ref : Inport
  vdq : Inport  Port=2
  idq : Inport  Port=3
  w_pu : Inport  Port=4
  1=-wLiq,+wLid_-1=+wLiq,-wLid : Inport  Port=5
  Add6 : Sum  Inputs=+++
  Add7 : Sum  Inputs=+-
  Add8 : Sum  Inputs=+++
  Add9 : Sum  Inputs=+-
  Bus Creator : BusCreator  Inputs=4
  Complex to Magnitude-Angle : ComplexToMagnitudeAngle
  Complex to Real-Imag : ComplexToRealImag
  Constant3 : Constant  Value=(1.0*Ts*fn*2*pi+TrafoPhaseComp)  SampleTime=Ts
  Constant6 : Constant  Value=-L  SampleTime=Ts
  Constant7 : Constant  Value=L  SampleTime=Ts
  Demux1 : Demux  Outputs=2
  Demux3 : Demux  Outputs=2
  Demux4 : Demux  Outputs=2
  Magnitude-Angle to Complex : MagnitudeAngleToComplex
  Mux2 : Mux  Inputs=2
  NotEqual : RelationalOperator  Operator=~=  OutDataTypeStr=boolean  RndMeth=Simplest
  NotEqual1 : RelationalOperator  Operator=~=  OutDataTypeStr=boolean  RndMeth=Simplest
  PI_id : $bdroot/Offshore_Oil_and_Wind/PI_Kp_Ti_AntiWindup  Ts=Ts  Kp=Kp  Ti=Ti  PI_max=PI_max  PI_min=PI_min
  PI_iq : $bdroot/Offshore_Oil_and_Wind/PI_Kp_Ti_AntiWindup  Ts=Ts  Kp=Kp  Ti=Ti  PI_max=PI_max  PI_min=PI_min
  Product1 : Product  RndMeth=Zero
  Product2 : Product  RndMeth=Zero
  Product6 : Product  Inputs=3  RndMeth=Zero
  Product7 : Product  Inputs=3  RndMeth=Zero
  Real-Imag to Complex : RealImagToComplex
  Relay : Relay  OnSwitchValue=0  OffSwitchValue=-0.1  OffOutputValue=-1
  Saturation1 : Saturate  UpperLimit=PI_max  LowerLimit=PI_min
  Saturation2 : Saturate  UpperLimit=PI_max  LowerLimit=PI_min
  Sum2 : Sum  Inputs=|++
  Terminator{,1..3} (4 alike) : Terminator
  Unit Delay1 : UnitDelay  SampleTime=Ts
  Unit Delay2 : UnitDelay  SampleTime=Ts
  vdq_ref : Outport
  m : Outport  Port=2
  wires:
  PI_iq/1 -> [PIq], Add8/2  "pi_iq"
  PI_iq/2 -> Terminator2/1
  PI_id/2 -> Terminator1/1
  w_pu/1 -> Product7/3, Product6/3
  Add9/1 -> PI_iq/1  "error"
  PI_id/1 -> [PId], Add6/2  "pi_id"
  Constant6/1 -> Product1/1
  Constant7/1 -> Product2/1
  Demux1/1 -> Add7/2, Product7/1  "id"
  Product7/1 -> [Q_decoup], Add8/3  "id_L_w"
  Demux4/1 -> Add6/1  "vd"
  Add7/1 -> PI_id/1  "error"
  Demux1/2 -> Product6/1, Add9/2  "iq"
  Product6/1 -> [D_decoup], Add6/3  "minus_iq_L_w"
  PI_iq/3 -> Terminator3/1
  PI_id/3 -> Terminator/1
  Demux4/2 -> Add8/1  "vq"
  Mux2/1 -> vdq_ref/1  "vdq_ref"
  idq/1 -> Demux1/1
  vdq/1 -> Demux4/1
  Add8/1 -> NotEqual1/1, Saturation2/1  "vq_ref"
  Add6/1 -> NotEqual/1, Saturation1/1  "vd_ref"
  idq_ref/1 -> Demux3/1
  Demux3/1 -> Add7/1  "idref"
  Demux3/2 -> Add9/1  "iqref"
  Magnitude-Angle to Complex/1 -> Complex to Real-Imag/1
  Real-Imag to Complex/1 -> Complex to Magnitude-Angle/1
  Complex to Magnitude-Angle/1 -> Magnitude-Angle to Complex/1
  Complex to Magnitude-Angle/2 -> Sum2/1
  Sum2/1 -> Magnitude-Angle to Complex/2
  Constant3/1 -> Sum2/2
  Complex to Real-Imag/1 -> Mux2/1
  Complex to Real-Imag/2 -> Mux2/2
  [PId] -> Bus Creator/1  "PI_D"
  [D_decoup] -> Bus Creator/2  "D_decoup"
  [PIq] -> Bus Creator/3  "PI_Q"
  Bus Creator/1 -> m/1
  [Q_decoup] -> Bus Creator/4  "Q_decoup"
  Saturation1/1 -> NotEqual/2, Real-Imag to Complex/1
  NotEqual/1 -> Unit Delay2/1
  Saturation2/1 -> NotEqual1/2, Real-Imag to Complex/2
  NotEqual1/1 -> Unit Delay1/1
  Unit Delay2/1 -> [dHold]
  Unit Delay1/1 -> [qHold]
  [dHold] -> PI_id/2
  [qHold] -> PI_iq/2
  Relay/1 -> [DecoupSign]
  1=-wLiq,+wLid_-1=+wLiq,-wLid/1 -> Relay/1
  [DecoupSign] -> Product1/2
  Product1/1 -> Product6/2
  Product2/1 -> Product7/2
  [DecoupSign] -> Product2/2

== system PhD_Library/Offshore_Oil_and_Wind/LSC_LCL_Trafo ==
  Gates : Inport
  Block_IGBTs : Inport  Port=2
  Open_Close_Breaker : Inport  Port=3
  Bus Creator : BusCreator  Inputs=8
  HV : powerlib/Measurements/Three-Phase V-I Measurement  VoltageMeasurement=phase-to-ground  SetLabelV=off  LabelV=vgrid  Vpu=off  VpuLL=off  CurrentMeasurement=yes  SetLabelI=off  LabelI=igrid  Ipu=off  Pbase=sn  Vbase=uab  OutputType=Complex  PhasorSimulation=off  PSBequivalent=0
  High Res Grounding : powerlib/Elements/Three-Phase Parallel RLC Load  LConnTagsString=A|B|C  Configuration=Y (grounded)  NominalVoltage=Uab  Vabc=[1e3 1e3 1e3]  Vabcp=[1e3 1e3 1e3]  NominalFrequency=fn  UnbalancedPower=off  ActivePower=0.001  InductivePower=0  CapacitivePower=0  Pabc=[10e3 9e3 11e3]  QLabc=[100 90 110]  QCabc=[100 90 110]  Pabcp=[10e3 9e3 11e3]  QLabcp=[100 90 110]  QCabcp=[100 90 110]  Measurements=None  LoadType=constant Z
  INV : powerlib/Measurements/Three-Phase V-I Measurement  VoltageMeasurement=phase-to-ground  SetLabelV=off  LabelV=vconv  Vpu=off  VpuLL=off  CurrentMeasurement=yes  SetLabelI=off  LabelI=iconv  Ipu=off  Pbase=sn  Vbase=uab  OutputType=Complex  PhasorSimulation=off  PSBequivalent=0
  INV_DClink : Subsystem
  LSC : powerlib/Power Electronics/Two-Level Converter  ModelType=Switching devices  Ron=1e-3  Rs=1e6  Cs=inf  Vforward=[ 0, 0 ]  Ron_Diode=1e-3  Rs_Diode=1e6  Cs_Diode=inf  Vf_Diode=1e-3  Rs_CurrentSource=inf
      settings: AttributesFormatString=%<ModelType>  SourceProductName=Simscape Power Systems  SourceProductBaseCode=PS
  LV : powerlib/Measurements/Three-Phase V-I Measurement  VoltageMeasurement=phase-to-ground  SetLabelV=off  LabelV=vgrid  Vpu=off  VpuLL=off  CurrentMeasurement=yes  SetLabelI=off  LabelI=igrid  Ipu=off  Pbase=sn  Vbase=uab  OutputType=Complex  PhasorSimulation=off  PSBequivalent=0
  La_DVR1 : powerlib/Elements/Series RLC Branch  LConnTagsString=__new0  RConnTagsString=__new0  BranchType=RL  Resistance=Rf1  Inductance=Lf1  SetiL0=off  InitialCurrent=0  Capacitance=1.0  Setx0=off  InitialVoltage=0  Measurements=None
  La_DVR2 : powerlib/Elements/Series RLC Branch  LConnTagsString=__new0  RConnTagsString=__new0  BranchType=RL  Resistance=Rf1  Inductance=Lf1  SetiL0=off  InitialCurrent=0  Capacitance=1.0  Setx0=off  InitialVoltage=0  Measurements=None
  La_DVR3 : powerlib/Elements/Series RLC Branch  LConnTagsString=__new0  RConnTagsString=__new0  BranchType=RL  Resistance=Rf1  Inductance=Lf1  SetiL0=off  InitialCurrent=0  Capacitance=1.0  Setx0=off  InitialVoltage=0  Measurements=None
  La_DVR4 : powerlib/Elements/Series RLC Branch  LConnTagsString=__new0  RConnTagsString=__new0  BranchType=RC  Resistance=Rc  Inductance=Lf1  SetiL0=off  InitialCurrent=0  Capacitance=Cf  Setx0=off  InitialVoltage=0  Measurements=None
  La_DVR5 : powerlib/Elements/Series RLC Branch  LConnTagsString=__new0  RConnTagsString=__new0  BranchType=RC  Resistance=Rc  Inductance=Lf1  SetiL0=off  InitialCurrent=0  Capacitance=Cf  Setx0=off  InitialVoltage=0  Measurements=None
  La_DVR6 : powerlib/Elements/Series RLC Branch  LConnTagsString=__new0  RConnTagsString=__new0  BranchType=RC  Resistance=Rc  Inductance=Lf1  SetiL0=off  InitialCurrent=0  Capacitance=Cf  Setx0=off  InitialVoltage=0  Measurements=None
  Three-Phase Transformer (Two Windings) : powerlib/Elements/Three-Phase Transformer (Two Windings)  Winding1Connection=Y  Winding2Connection=Delta (D1)  CoreType=Three-limb core (core-type)  SetSaturation=off  Hysteresis=off  DataFile='hysteresis'  SetInitialFlux=off  Measurements=None  UNITS=pu  NominalPower=[ Sn , fn ]  Winding1=[ Uhv_ab , rf2/2 , lf2/2 ]  Winding2=[ Uab , rf2/2 , lf2/2 ]  Rm=500  Lm=500  L0=0.5  Saturation=[ 0,0 ; 0.0024,1.2 ; 1.0,1.52 ]  InitialFluxes=[0 0 0]  MoreParameters=off  BreakLoop=off  DataType=off  TransfoNumber=1
  Three-Phase Breaker : powerlib/Elements/Three-Phase Breaker  InitialState=open  SwitchA=on  SwitchB=on  SwitchC=on  SwitchTimes="[1/60  5/60]"  External=on  BreakerResistance=0.01  SnubberResistance=1e6  SnubberCapacitance=inf  Measurements=None
  "\tP" : PMIOPort  Side=Left
  M : PMIOPort  Port=2  Side=Left
  A : PMIOPort  Port=3  Side=Right
  B : PMIOPort  Port=4  Side=Right
  C : PMIOPort  Port=5  Side=Right
  m : Outport
  wires:
  HV/2 -> Bus Creator/2  "HV_Iabc"
  LV/1 -> Bus Creator/3  "LV_Vabc"
  INV/1 -> Bus Creator/5  "INV_Vabc"
  INV_DClink/2(Idc) -> Bus Creator/8  "Idc"
  INV/2 -> Bus Creator/6  "INV_Iabc"
  Block_IGBTs/1 -> LSC/2
  INV_DClink/1(Vdc) -> Bus Creator/7  "Vdc"
  HV/1 -> Bus Creator/1  "HV_Vabc"
  LV/2 -> Bus Creator/4  "LV_Iabc"
  Bus Creator/1 -> m/1
  Gates/1 -> LSC/1
  Open_Close_Breaker/1 -> Three-Phase Breaker/1
  connections:
  La_DVR1/LConn1 -- INV/RConn1
  LV/RConn1 -- Three-Phase Transformer (Two Windings)/RConn1 -- High Res Grounding/LConn1
  La_DVR1/RConn1 -- La_DVR4/RConn1 -- LV/LConn1
  LSC/LConn3 -- INV/LConn3
  Three-Phase Transformer (Two Windings)/LConn3 -- HV/LConn3
  LSC/LConn2 -- INV/LConn2
  Three-Phase Transformer (Two Windings)/RConn3 -- LV/RConn3 -- High Res Grounding/LConn3
  La_DVR2/RConn1 -- La_DVR5/RConn1 -- LV/LConn2
  Three-Phase Transformer (Two Windings)/LConn2 -- HV/LConn2
  LSC/RConn2 -- INV_DClink/RConn2
  LSC/LConn1 -- INV/LConn1
  LSC/RConn1 -- INV_DClink/RConn1
  Three-Phase Transformer (Two Windings)/RConn2 -- LV/RConn2 -- High Res Grounding/LConn2
  "\tP"/RConn1 -- INV_DClink/LConn1
  Three-Phase Transformer (Two Windings)/LConn1 -- HV/LConn1
  LV/LConn3 -- La_DVR3/RConn1 -- La_DVR6/RConn1
  La_DVR3/LConn1 -- INV/RConn3
  La_DVR5/LConn1 -- La_DVR6/LConn1 -- La_DVR4/LConn1
  La_DVR2/LConn1 -- INV/RConn2
  INV_DClink/LConn2 -- M/RConn1
  Three-Phase Breaker/LConn2 -- B/RConn1
  Three-Phase Breaker/RConn2 -- HV/RConn2
  HV/RConn3 -- Three-Phase Breaker/RConn3
  Three-Phase Breaker/LConn3 -- C/RConn1
  HV/RConn1 -- Three-Phase Breaker/RConn1
  Three-Phase Breaker/LConn1 -- A/RConn1

== system PhD_Library/Offshore_Oil_and_Wind/LSC_LCL_Trafo_AvgxSwitch ==
  Gates : Inport
  0=Avg_1=Switch : Inport  Port=2
  Open_Close_Breaker : Inport  Port=3
  Vabcref : Inport  Port=4
  Bus Creator : BusCreator  Inputs=8
  Constant : Constant  Value=0
  Constant1 : Constant  Value=0
  Constant2 : Constant
  Constant3 : Constant
  Constant4 : Constant  Value=0
  Controlled Voltage Source : powerlib/Electrical Sources/Controlled Voltage Source  Initialize=off  Source_Type=AC  Amplitude=ESS.LSC.Ub*(2/3)^0.5  Phase=0  Frequency=PCC.fn  Measurements=None
  Controlled Voltage Source1 : powerlib/Electrical Sources/Controlled Voltage Source  Initialize=off  Source_Type=AC  Amplitude=ESS.LSC.Ub*(2/3)^0.5  Phase=-120  Frequency=PCC.fn  Measurements=None
  Controlled Voltage Source2 : powerlib/Electrical Sources/Controlled Voltage Source  Initialize=off  Source_Type=AC  Amplitude=ESS.LSC.Ub*(2/3)^0.5  Phase=120  Frequency=PCC.fn  Measurements=None
  Demux2 : Demux  Outputs=3
  HV : powerlib/Measurements/Three-Phase V-I Measurement  VoltageMeasurement=phase-to-ground  SetLabelV=off  LabelV=vgrid  Vpu=off  VpuLL=off  CurrentMeasurement=yes  SetLabelI=off  LabelI=igrid  Ipu=off  Pbase=sn  Vbase=uab  OutputType=Complex  PhasorSimulation=off  PSBequivalent=0
  High Res Grounding : powerlib/Elements/Three-Phase Parallel RLC Load  LConnTagsString=A|B|C  Configuration=Y (grounded)  NominalVoltage=Uab  Vabc=[1e3 1e3 1e3]  Vabcp=[1e3 1e3 1e3]  NominalFrequency=fn  UnbalancedPower=off  ActivePower=0.001  InductivePower=0  CapacitivePower=0  Pabc=[10e3 9e3 11e3]  QLabc=[100 90 110]  QCabc=[100 90 110]  Pabcp=[10e3 9e3 11e3]  QLabcp=[100 90 110]  QCabcp=[100 90 110]  Measurements=None  LoadType=constant Z
  INV : powerlib/Measurements/Three-Phase V-I Measurement  VoltageMeasurement=phase-to-ground  SetLabelV=off  LabelV=vconv  Vpu=off  VpuLL=off  CurrentMeasurement=yes  SetLabelI=off  LabelI=iconv  Ipu=off  Pbase=sn  Vbase=uab  OutputType=Complex  PhasorSimulation=off  PSBequivalent=0
  INV_DClink : Subsystem
  LSC : powerlib/Power Electronics/Two-Level Converter  ModelType=Switching devices  Ron=1e-3  Rs=1e6  Cs=inf  Vforward=[ 0, 0 ]  Ron_Diode=1e-3  Rs_Diode=1e6  Cs_Diode=inf  Vf_Diode=1e-3  Rs_CurrentSource=inf
      settings: AttributesFormatString=%<ModelType>  SourceProductName=Simscape Power Systems  SourceProductBaseCode=PS
  LV : powerlib/Measurements/Three-Phase V-I Measurement  VoltageMeasurement=phase-to-ground  SetLabelV=off  LabelV=vgrid  Vpu=off  VpuLL=off  CurrentMeasurement=yes  SetLabelI=off  LabelI=igrid  Ipu=off  Pbase=sn  Vbase=uab  OutputType=Complex  PhasorSimulation=off  PSBequivalent=0
  La_DVR1 : powerlib/Elements/Series RLC Branch  LConnTagsString=__new0  RConnTagsString=__new0  BranchType=RL  Resistance=Rf1  Inductance=Lf1  SetiL0=off  InitialCurrent=0  Capacitance=1.0  Setx0=off  InitialVoltage=0  Measurements=None
  La_DVR2 : powerlib/Elements/Series RLC Branch  LConnTagsString=__new0  RConnTagsString=__new0  BranchType=RL  Resistance=Rf1  Inductance=Lf1  SetiL0=off  InitialCurrent=0  Capacitance=1.0  Setx0=off  InitialVoltage=0  Measurements=None
  La_DVR3 : powerlib/Elements/Series RLC Branch  LConnTagsString=__new0  RConnTagsString=__new0  BranchType=RL  Resistance=Rf1  Inductance=Lf1  SetiL0=off  InitialCurrent=0  Capacitance=1.0  Setx0=off  InitialVoltage=0  Measurements=None
  La_DVR4 : powerlib/Elements/Series RLC Branch  LConnTagsString=__new0  RConnTagsString=__new0  BranchType=RC  Resistance=Rc  Inductance=Lf1  SetiL0=off  InitialCurrent=0  Capacitance=Cf  Setx0=off  InitialVoltage=0  Measurements=None
  La_DVR5 : powerlib/Elements/Series RLC Branch  LConnTagsString=__new0  RConnTagsString=__new0  BranchType=RC  Resistance=Rc  Inductance=Lf1  SetiL0=off  InitialCurrent=0  Capacitance=Cf  Setx0=off  InitialVoltage=0  Measurements=None
  La_DVR6 : powerlib/Elements/Series RLC Branch  LConnTagsString=__new0  RConnTagsString=__new0  BranchType=RC  Resistance=Rc  Inductance=Lf1  SetiL0=off  InitialCurrent=0  Capacitance=Cf  Setx0=off  InitialVoltage=0  Measurements=None
  Switch : Switch  Criteria=u2 > Threshold  Threshold=0.5
  Switch1 : Switch  Criteria=u2 > Threshold  Threshold=0.5
  Three-Phase Transformer (Two Windings) : powerlib/Elements/Three-Phase Transformer (Two Windings)  Winding1Connection=Y  Winding2Connection=Delta (D1)  CoreType=Three-limb core (core-type)  SetSaturation=off  Hysteresis=off  DataFile='hysteresis'  SetInitialFlux=off  Measurements=None  UNITS=pu  NominalPower=[ Sn , fn ]  Winding1=[ Uhv_ab , rf2/2 , lf2/2 ]  Winding2=[ Uab , rf2/2 , lf2/2 ]  Rm=500  Lm=500  L0=0.5  Saturation=[ 0,0 ; 0.0024,1.2 ; 1.0,1.52 ]  InitialFluxes=[0 0 0]  MoreParameters=off  BreakLoop=off  DataType=off  TransfoNumber=1
  Three-Phase Breaker : powerlib/Elements/Three-Phase Breaker  InitialState=open  SwitchA=on  SwitchB=on  SwitchC=on  SwitchTimes="[1/60  5/60]"  External=on  BreakerResistance=0.01  SnubberResistance=1e6  SnubberCapacitance=inf  Measurements=None
  Three-Phase Breaker1 : powerlib/Elements/Three-Phase Breaker  InitialState=open  SwitchA=on  SwitchB=on  SwitchC=on  SwitchTimes="[1/60  5/60]"  External=on  BreakerResistance=0.000000000001  SnubberResistance=1e10  SnubberCapacitance=inf  Measurements=None
  Three-Phase Breaker2 : powerlib/Elements/Three-Phase Breaker  InitialState=open  SwitchA=on  SwitchB=on  SwitchC=on  SwitchTimes="[1/60  5/60]"  External=on  BreakerResistance=0.000000000001  SnubberResistance=1e10  SnubberCapacitance=inf  Measurements=None
  "\tP" : PMIOPort  Side=Left
  M : PMIOPort  Port=2  Side=Left
  A : PMIOPort  Port=3  Side=Right
  B : PMIOPort  Port=4  Side=Right
  C : PMIOPort  Port=5  Side=Right
  m : Outport
  wires:
  HV/2 -> Bus Creator/2  "HV_Iabc"
  LV/1 -> Bus Creator/3  "LV_Vabc"
  INV/1 -> Bus Creator/5  "INV_Vabc"
  INV_DClink/2(Idc) -> Bus Creator/8  "Idc"
  INV/2 -> Bus Creator/6  "INV_Iabc"
  INV_DClink/1(Vdc) -> Bus Creator/7  "Vdc"
  HV/1 -> Bus Creator/1  "HV_Vabc"
  LV/2 -> Bus Creator/4  "LV_Iabc"
  Bus Creator/1 -> m/1
  Gates/1 -> LSC/1
  Open_Close_Breaker/1 -> Three-Phase Breaker/1
  Vabcref/1 -> Demux2/1
  Demux2/1 -> Controlled Voltage Source/1  "Va"
  Demux2/2 -> Controlled Voltage Source1/1  "Vb"
  Demux2/3 -> Controlled Voltage Source2/1  "Vc"
  Constant/1 -> LSC/2
  Constant1/1 -> Switch/3
  Constant2/1 -> Switch/1
  Switch/1 -> Three-Phase Breaker1/1
  Constant4/1 -> Switch1/1
  Constant3/1 -> Switch1/3
  Switch1/1 -> Three-Phase Breaker2/1
  0=Avg_1=Switch/1 -> Switch1/2, Switch/2
  connections:
  La_DVR1/LConn1 -- INV/RConn1
  LV/RConn1 -- Three-Phase Transformer (Two Windings)/RConn1 -- High Res Grounding/LConn1
  La_DVR1/RConn1 -- La_DVR4/RConn1 -- LV/LConn1
  LSC/LConn3 -- Three-Phase Breaker1/RConn3
  Three-Phase Transformer (Two Windings)/LConn3 -- HV/LConn3
  LSC/LConn2 -- Three-Phase Breaker1/RConn2
  Three-Phase Transformer (Two Windings)/RConn3 -- LV/RConn3 -- High Res Grounding/LConn3
  La_DVR2/RConn1 -- La_DVR5/RConn1 -- LV/LConn2
  Three-Phase Transformer (Two Windings)/LConn2 -- HV/LConn2
  LSC/RConn2 -- INV_DClink/RConn2
  LSC/LConn1 -- Three-Phase Breaker1/RConn1
  LSC/RConn1 -- INV_DClink/RConn1
  Three-Phase Transformer (Two Windings)/RConn2 -- LV/RConn2 -- High Res Grounding/LConn2
  "\tP"/RConn1 -- INV_DClink/LConn1
  Three-Phase Transformer (Two Windings)/LConn1 -- HV/LConn1
  LV/LConn3 -- La_DVR3/RConn1 -- La_DVR6/RConn1
  La_DVR3/LConn1 -- INV/RConn3
  La_DVR5/LConn1 -- La_DVR6/LConn1 -- La_DVR4/LConn1
  La_DVR2/LConn1 -- INV/RConn2
  INV_DClink/LConn2 -- M/RConn1
  Three-Phase Breaker/LConn2 -- B/RConn1
  Three-Phase Breaker/RConn2 -- HV/RConn2
  HV/RConn3 -- Three-Phase Breaker/RConn3
  Three-Phase Breaker/LConn3 -- C/RConn1
  HV/RConn1 -- Three-Phase Breaker/RConn1
  Three-Phase Breaker/LConn1 -- A/RConn1
  Controlled Voltage Source2/LConn1 -- Controlled Voltage Source/LConn1 -- Controlled Voltage Source1/LConn1
  Three-Phase Breaker1/LConn1 -- Three-Phase Breaker2/LConn1 -- INV/LConn1
  Three-Phase Breaker1/LConn2 -- Three-Phase Breaker2/LConn2 -- INV/LConn2
  Three-Phase Breaker1/LConn3 -- Three-Phase Breaker2/LConn3 -- INV/LConn3
  Three-Phase Breaker2/RConn1 -- Controlled Voltage Source/RConn1
  Controlled Voltage Source1/RConn1 -- Three-Phase Breaker2/RConn2
  Controlled Voltage Source2/RConn1 -- Three-Phase Breaker2/RConn3
